simulink subsystem "STR"  (R2025b)
settings: Solver=VariableStepAuto  StartTime=0.0  StopTime=10.0  RelTol=1e-3
model mask{strUpdateFreq=0, strNoisePerChannel=0, strBiasPerChannel=0, strNoiseSeed=0}
  mask prompts: strUpdateFreq "Update frequency [Hz]"; strNoisePerChannel "Noise (3 sigma) [º]"; strBiasPerChannel "Bias [º]"; strNoiseSeed "Noise seeds"
settings Model: Creator=antoniohernandez-rodiciomateos  LastModifiedBy=antoniohernandez-rodiciomateos

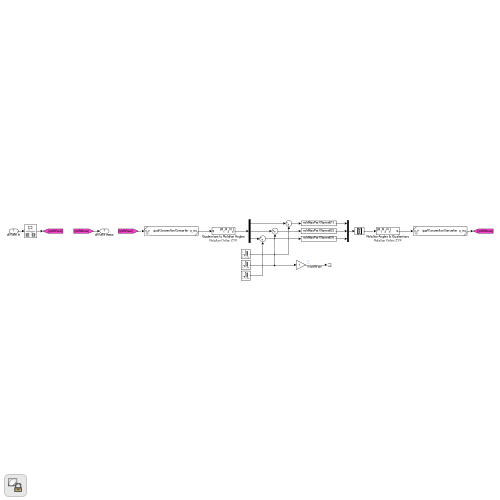
[thumbnail: Simulink's stored preview of the top-level diagram]
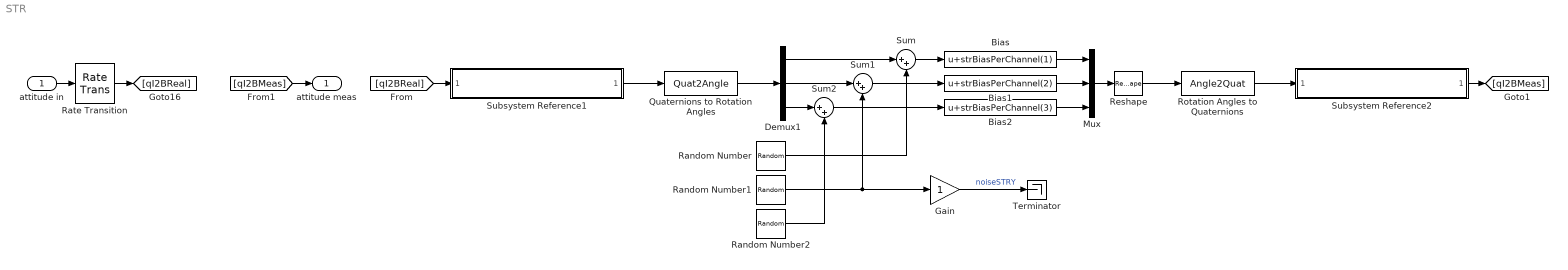
== system STR ==
  attitude in : Inport  OutDataTypeStr=double  PortDimensions=[4 1]
  Bias : Bias  Bias=strBiasPerChannel(1)  SaturateOnIntegerOverflow=off
  Bias1 : Bias  Bias=strBiasPerChannel(2)  SaturateOnIntegerOverflow=off
  Bias2 : Bias  Bias=strBiasPerChannel(3)  SaturateOnIntegerOverflow=off
  Demux1 : Demux  Outputs=3
  Gain : Gain
  Mux : Mux  Inputs=3
  Quaternions to Rotation Angles : Quat2Angle
      settings: AttributesFormatString=Rotation Order: %<rotationOrder>
  Random Number : RandomNumber  Variance=(strNoisePerChannel ^ 2) / 9  Seed=strNoiseSeed(1)  SampleTime=1 / strUpdateFreq
  Random Number1 : RandomNumber  Variance=(strNoisePerChannel ^ 2) / 9  Seed=strNoiseSeed(2)  SampleTime=1 / strUpdateFreq
  Random Number2 : RandomNumber  Variance=(strNoisePerChannel ^ 2) / 9  Seed=strNoiseSeed(3)  SampleTime=1 / strUpdateFreq
  Rate Transition : RateTransition  OutPortSampleTime=1 / strUpdateFreq
  Reshape : Reshape  OutputDimensionality=Column vector (2-D)
  Rotation Angles to Quaternions : Angle2Quat
      settings: AttributesFormatString=Rotation Order: %<rotationOrder>
  Subsystem Reference1 : Subsystem  ReferencedSubsystem=quatConventionConverter  conversion=q4 to q0
  Subsystem Reference2 : Subsystem  ReferencedSubsystem=quatConventionConverter  conversion=q0 to q4
  Sum : Sum  Inputs=|++
  Sum1 : Sum  Inputs=|++
  Sum2 : Sum  Inputs=|++
  Terminator : Terminator
  attitude meas : Outport  OutDataTypeStr=double  PortDimensions=[4 1]
  wires:
  [qI2BReal] -> Subsystem Reference1/1
  Subsystem Reference1/1 -> Quaternions to Rotation Angles/1
  Demux1/1 -> Sum/1
  Mux/1 -> Reshape/1
  Demux1/3 -> Sum2/1
  Quaternions to Rotation Angles/1 -> Demux1/1
  Random Number2/1 -> Sum2/2
  Random Number1/1 -> Sum1/2, Gain/1
  Random Number/1 -> Sum/2
  Demux1/2 -> Sum1/1
  Reshape/1 -> Rotation Angles to Quaternions/1
  Rotation Angles to Quaternions/1 -> Subsystem Reference2/1
  Sum/1 -> Bias/1
  Bias/1 -> Mux/1
  Sum1/1 -> Bias1/1
  Sum2/1 -> Bias2/1
  Bias1/1 -> Mux/2
  Bias2/1 -> Mux/3
  [qI2BMeas] -> attitude meas/1
  Subsystem Reference2/1 -> [qI2BMeas]
  Gain/1 -> Terminator/1  "noiseSTRY"
  attitude in/1 -> Rate Transition/1
  Rate Transition/1 -> [qI2BReal]
